simulink model "Tesis_Rectificador_Controlador_Observador_04"  (R2012b)
settings: Solver=ode1  StartTime=0.0  StopTime=1.0  FixedStep=1e-5/6  RelTol=1e-3
libraries: simulink x1
settings Model: Creator=Ramm  LastModifiedBy=Ramm

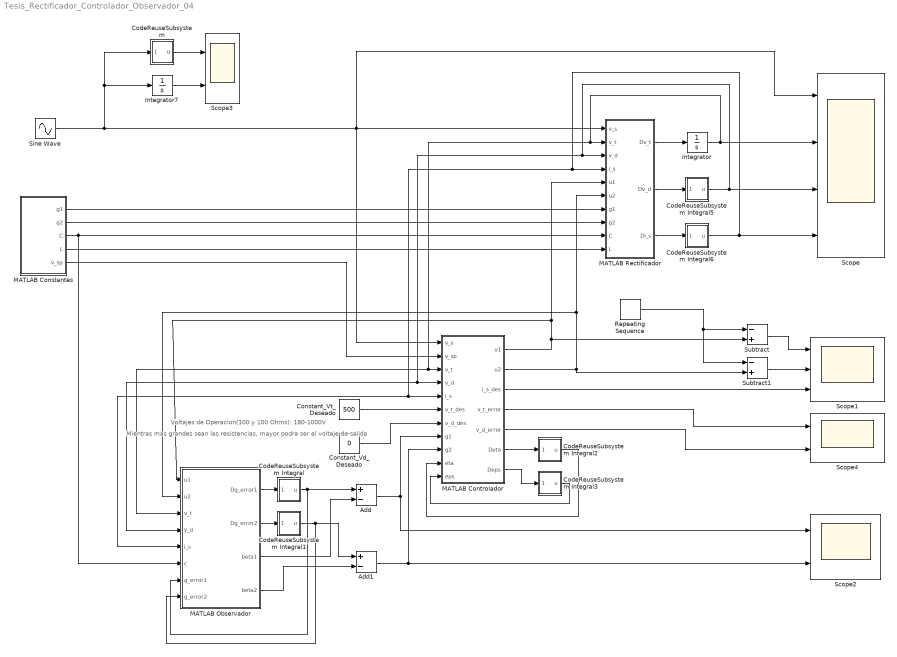
== system Tesis_Rectificador_Controlador_Observador_04 ==
  note: Mientras mas grandes sean las resistencias,
      | mayor podra ser el voltaje de salida
  note: Voltajes de Operacion(100 y 100 Ohms): 180-1000V
  Add : Sum  Inputs=+-
  Add1 : Sum  Inputs=+-
  CodeReuseSubsystem : Subsystem  TreatAsAtomicUnit=on
      settings: RTWFcnNameOpts=Use subsystem name  RTWFileNameOpts=Use function name
  CodeReuseSubsystem Integral : Subsystem  TreatAsAtomicUnit=on
      settings: RTWFcnNameOpts=Use subsystem name  RTWFileNameOpts=Use function name
  CodeReuseSubsystem Integral1 : Subsystem  TreatAsAtomicUnit=on
      settings: RTWFcnNameOpts=Use subsystem name  RTWFileNameOpts=Use function name
  CodeReuseSubsystem Integral2 : Subsystem  TreatAsAtomicUnit=on
      settings: RTWFcnNameOpts=Use subsystem name  RTWFileNameOpts=Use function name
  CodeReuseSubsystem Integral3 : Subsystem  TreatAsAtomicUnit=on
      settings: RTWFcnNameOpts=Use subsystem name  RTWFileNameOpts=Use function name
  CodeReuseSubsystem Integral5 : Subsystem  TreatAsAtomicUnit=on
      settings: RTWFcnNameOpts=Use subsystem name  RTWFileNameOpts=Use function name
  CodeReuseSubsystem Integral6 : Subsystem  TreatAsAtomicUnit=on
      settings: RTWFcnNameOpts=Use subsystem name  RTWFileNameOpts=Use function name
  Constant_Vd_Deseado : Constant  Value=0
  Constant_Vt_Deseado : Constant  Value=500
  Integrator : Integrator
  Integrator7 : Integrator  InitialCondition=0.02
  "MATLAB Constantes " : MATLAB Function  TreatAsAtomicUnit=on
  MATLAB Controlador : MATLAB Function  TreatAsAtomicUnit=on
  "MATLAB Observador " : MATLAB Function  TreatAsAtomicUnit=on
  "MATLAB Rectificador " : MATLAB Function  TreatAsAtomicUnit=on
  Repeating Sequence : simulink/Sources/Repeating Sequence  rep_seq_t=[0 1.655e-5]  rep_seq_y=[0 1]
  Scope : Scope  NumInputPorts=4
      settings: TimeRange=0.5  YMin=-200~425~-1.525~-30  YMax=200~600~-1.325~25
  Scope1 : Scope  NumInputPorts=3
      settings: TimeRange=1  YMin=-350~-350~-1.5  YMax=350~350~1.5
  Scope2 : Scope  NumInputPorts=2
      settings: TimeRange=0.7000000000000001  YMin=-0.002~-0.005  YMax=0.012~0.02  SaveName=ScopeData3
  Scope3 : Scope  NumInputPorts=2
      settings: YMin=-5~-5  YMax=5~5  SaveName=ScopeData4
  Scope4 : Scope  NumInputPorts=2
      settings: YMin=-129~-1.035  YMax=-118~-0.945  SaveName=ScopeData2
  Sine Wave : Sin  Amplitude=180  Frequency=120*pi  SampleTime=0
  Subtract : Sum  Inputs=-+
  Subtract1 : Sum  Inputs=-+
  wires:
  Constant_Vt_Deseado/1 -> MATLAB Controlador/6(v_t_des)
  Constant_Vd_Deseado/1 -> MATLAB Controlador/7(v_d_des)
  "MATLAB Observador "/1(Dg_error1) -> CodeReuseSubsystem Integral/1(Du)
  CodeReuseSubsystem Integral/1(u) -> "MATLAB Observador "/7(g_error1), Add/1
  Add/1 -> Scope2/1, MATLAB Controlador/8(g1)
  Add1/1 -> MATLAB Controlador/9(g2), Scope2/2
  MATLAB Controlador/6(Deta) -> CodeReuseSubsystem Integral2/1(Du)
  MATLAB Controlador/7(Deps) -> CodeReuseSubsystem Integral3/1(Du)
  CodeReuseSubsystem Integral2/1(u) -> MATLAB Controlador/10(eta)
  CodeReuseSubsystem Integral3/1(u) -> MATLAB Controlador/11(eps)
  "MATLAB Constantes "/1(g1) -> "MATLAB Rectificador "/7(g1)
  "MATLAB Constantes "/2(g2) -> "MATLAB Rectificador "/8(g2)
  "MATLAB Constantes "/3(C) -> "MATLAB Observador "/6(c), "MATLAB Rectificador "/9(C)
  "MATLAB Constantes "/4(L) -> "MATLAB Rectificador "/10(L)
  "MATLAB Constantes "/5(v_sp) -> MATLAB Controlador/2(v_sp)
  Sine Wave/1 -> CodeReuseSubsystem/1(Du), Integrator7/1, Scope/1, MATLAB Controlador/1(v_s), "MATLAB Rectificador "/1(v_s)
  "MATLAB Rectificador "/1(Dv_t) -> Integrator/1
  "MATLAB Rectificador "/2(Dv_d) -> CodeReuseSubsystem Integral5/1(Du)
  "MATLAB Rectificador "/3(Di_s) -> CodeReuseSubsystem Integral6/1(Du)
  MATLAB Controlador/1(u1) -> Subtract/2, "MATLAB Observador "/1(u1), "MATLAB Rectificador "/5(u1)
  Integrator/1 -> Scope/2, "MATLAB Observador "/3(v_t), MATLAB Controlador/3(v_t), "MATLAB Rectificador "/2(v_t)
  CodeReuseSubsystem Integral5/1(u) -> Scope/3, MATLAB Controlador/4(v_d), "MATLAB Observador "/4(v_d), "MATLAB Rectificador "/3(v_d)
  CodeReuseSubsystem Integral6/1(u) -> Scope/4, "MATLAB Observador "/5(i_s), MATLAB Controlador/5(i_s), "MATLAB Rectificador "/4(i_s)
  MATLAB Controlador/4(v_t_error) -> Scope4/1
  MATLAB Controlador/5(v_d_error) -> Scope4/2
  MATLAB Controlador/3(i_s_des) -> Scope1/3
  "MATLAB Observador "/3(beta1) -> Add/2
  "MATLAB Observador "/2(Dg_error2) -> CodeReuseSubsystem Integral1/1(Du)
  CodeReuseSubsystem Integral1/1(u) -> "MATLAB Observador "/8(g_error2), Add1/1
  "MATLAB Observador "/4(beta2) -> Add1/2
  MATLAB Controlador/2(u2) -> "MATLAB Rectificador "/6(u2), "MATLAB Observador "/2(u2), Subtract1/2
  Subtract1/1 -> Scope1/2
  Subtract/1 -> Scope1/1
  Repeating Sequence/1 -> Subtract/1, Subtract1/1
  CodeReuseSubsystem/1(u) -> Scope3/1
  Integrator7/1 -> Scope3/2

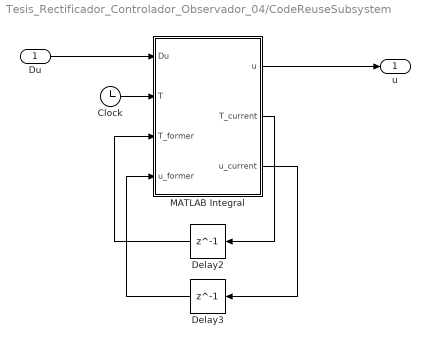
== system Tesis_Rectificador_Controlador_Observador_04/CodeReuseSubsystem ==
  Du : Inport
  Clock : Clock
  Delay2 : Delay  DelayLength=1  InitialCondition=0
  Delay3 : Delay  DelayLength=1  InitialCondition=0
  MATLAB Integral : MATLAB Function  TreatAsAtomicUnit=on
  u : Outport
  wires:
  Clock/1 -> MATLAB Integral/2(T)
  Du/1 -> MATLAB Integral/1(Du)
  MATLAB Integral/1(u) -> u/1
  Delay3/1 -> MATLAB Integral/4(u_former)
  MATLAB Integral/3(u_current) -> Delay3/1
  Delay2/1 -> MATLAB Integral/3(T_former)
  MATLAB Integral/2(T_current) -> Delay2/1

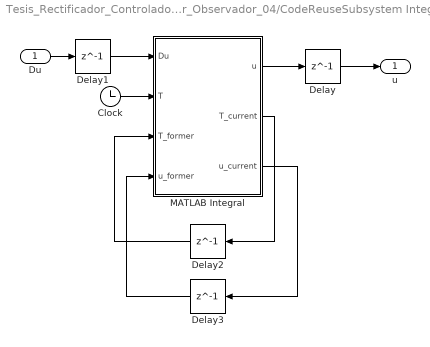
== system Tesis_Rectificador_Controlador_Observador_04/CodeReuseSubsystem Integral ==
  Du : Inport
  Clock : Clock
  Delay{,1..3} (4 alike) : Delay  DelayLength=1  InitialCondition=0
  MATLAB Integral : MATLAB Function  TreatAsAtomicUnit=on
  u : Outport
  wires:
  MATLAB Integral/2(T_current) -> Delay2/1
  Delay2/1 -> MATLAB Integral/3(T_former)
  MATLAB Integral/3(u_current) -> Delay3/1
  Delay3/1 -> MATLAB Integral/4(u_former)
  Clock/1 -> MATLAB Integral/2(T)
  MATLAB Integral/1(u) -> Delay/1
  Delay/1 -> u/1
  Du/1 -> Delay1/1
  Delay1/1 -> MATLAB Integral/1(Du)

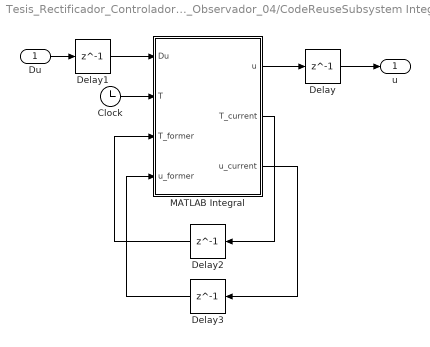
== system Tesis_Rectificador_Controlador_Observador_04/CodeReuseSubsystem Integral1 ==
  Du : Inport
  Clock : Clock
  Delay{,1..3} (4 alike) : Delay  DelayLength=1  InitialCondition=0
  MATLAB Integral : MATLAB Function  TreatAsAtomicUnit=on
  u : Outport
  wires:
  Delay1/1 -> MATLAB Integral/1(Du)
  Du/1 -> Delay1/1
  Delay/1 -> u/1
  MATLAB Integral/1(u) -> Delay/1
  Clock/1 -> MATLAB Integral/2(T)
  Delay3/1 -> MATLAB Integral/4(u_former)
  MATLAB Integral/3(u_current) -> Delay3/1
  Delay2/1 -> MATLAB Integral/3(T_former)
  MATLAB Integral/2(T_current) -> Delay2/1

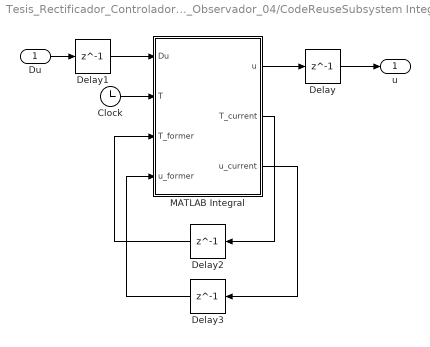
== system Tesis_Rectificador_Controlador_Observador_04/CodeReuseSubsystem Integral2 ==
  Du : Inport
  Clock : Clock
  Delay{,1..3} (4 alike) : Delay  DelayLength=1  InitialCondition=0
  MATLAB Integral : MATLAB Function  TreatAsAtomicUnit=on
  u : Outport
  wires:
  MATLAB Integral/2(T_current) -> Delay2/1
  Delay2/1 -> MATLAB Integral/3(T_former)
  MATLAB Integral/3(u_current) -> Delay3/1
  Delay3/1 -> MATLAB Integral/4(u_former)
  Clock/1 -> MATLAB Integral/2(T)
  MATLAB Integral/1(u) -> Delay/1
  Delay/1 -> u/1
  Du/1 -> Delay1/1
  Delay1/1 -> MATLAB Integral/1(Du)

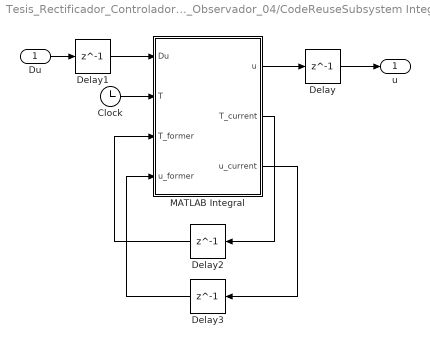
== system Tesis_Rectificador_Controlador_Observador_04/CodeReuseSubsystem Integral3 ==
  Du : Inport
  Clock : Clock
  Delay{,1..3} (4 alike) : Delay  DelayLength=1  InitialCondition=0
  MATLAB Integral : MATLAB Function  TreatAsAtomicUnit=on
  u : Outport
  wires:
  Delay1/1 -> MATLAB Integral/1(Du)
  Du/1 -> Delay1/1
  Delay/1 -> u/1
  MATLAB Integral/1(u) -> Delay/1
  Clock/1 -> MATLAB Integral/2(T)
  Delay3/1 -> MATLAB Integral/4(u_former)
  MATLAB Integral/3(u_current) -> Delay3/1
  Delay2/1 -> MATLAB Integral/3(T_former)
  MATLAB Integral/2(T_current) -> Delay2/1

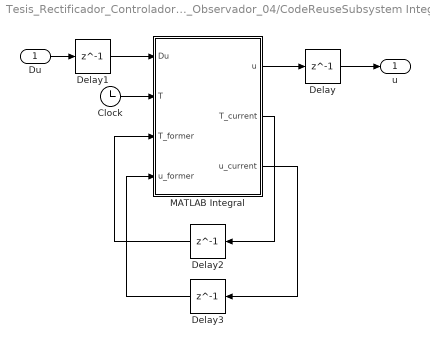
== system Tesis_Rectificador_Controlador_Observador_04/CodeReuseSubsystem Integral5 ==
  Du : Inport
  Clock : Clock
  Delay : Delay  DelayLength=1  InitialCondition=1
  Delay1 : Delay  DelayLength=1  InitialCondition=0
  Delay2 : Delay  DelayLength=1  InitialCondition=0
  Delay3 : Delay  DelayLength=1  InitialCondition=0
  MATLAB Integral : MATLAB Function  TreatAsAtomicUnit=on
  u : Outport
  wires:
  Delay1/1 -> MATLAB Integral/1(Du)
  Du/1 -> Delay1/1
  Delay/1 -> u/1
  MATLAB Integral/1(u) -> Delay/1
  Clock/1 -> MATLAB Integral/2(T)
  Delay3/1 -> MATLAB Integral/4(u_former)
  MATLAB Integral/3(u_current) -> Delay3/1
  Delay2/1 -> MATLAB Integral/3(T_former)
  MATLAB Integral/2(T_current) -> Delay2/1

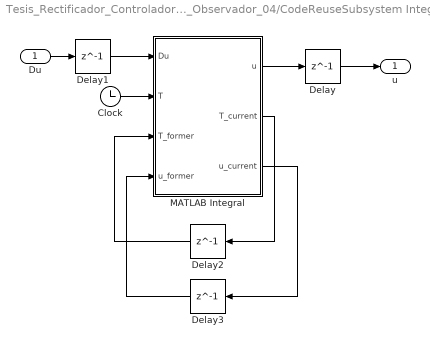
== system Tesis_Rectificador_Controlador_Observador_04/CodeReuseSubsystem Integral6 ==
  Du : Inport
  Clock : Clock
  Delay : Delay  DelayLength=1  InitialCondition=1
  Delay1 : Delay  DelayLength=1  InitialCondition=0
  Delay2 : Delay  DelayLength=1  InitialCondition=0
  Delay3 : Delay  DelayLength=1  InitialCondition=0
  MATLAB Integral : MATLAB Function  TreatAsAtomicUnit=on
  u : Outport
  wires:
  MATLAB Integral/2(T_current) -> Delay2/1
  Delay2/1 -> MATLAB Integral/3(T_former)
  MATLAB Integral/3(u_current) -> Delay3/1
  Delay3/1 -> MATLAB Integral/4(u_former)
  Clock/1 -> MATLAB Integral/2(T)
  MATLAB Integral/1(u) -> Delay/1
  Delay/1 -> u/1
  Du/1 -> Delay1/1
  Delay1/1 -> MATLAB Integral/1(Du)

== matlab function Tesis_Rectificador_Controlador_Observador_04/MATLAB Controlador ==
  data: v_s input; v_sp input; u1 output; v_t input; v_d input; i_s input; v_t_des input; v_d_des input; g1 input; g2 input; u2 output; i_s_des output; v_t_error output; v_d_error output; Deta output; Deps output; eta input; eps input
function [u1, u2, i_s_des, v_t_error, v_d_error, Deta, Deps] = fcn(v_s, v_sp, v_t, v_d, i_s, v_t_des, v_d_des, g1, g2, eta, eps)
%#codegen
%Constantes de proporcionalidad -----------------------------------
k = 10000;%Se encarga de disminuir el error de la corriente, mientras mas grande sea mas rapido decaera el error, pero puede volverse inestable

%Para la corriente deseada
kp1 = 1e-2;%1e-2;%Debe ser muy chico para ver el observador pero deja de controlar(Oscilatorio (v_t))
ki1 = 10;%1e-2;%Debe ser muy chico para ver el observador pero deja de controlar(Compensacion de estado estable(v_t))

%Señales de control
kp2 = 250;%250;
ki2 = 500;%500;

%*****************************************************************************************************************************
%Calculos previos-------------------------------------------------
v_t_error = v_t - v_t_des;
i_s_des = -((v_s*v_t)/(2*v_sp*v_sp))*(-g1*v_t -g2*v_d + kp1*v_t_error +ki1*eta);
i_s_error = i_s - i_s_des;
v_d_error = v_d - v_d_des;

%Salidas-------------------------------------------------

%Con los despejes hechos previamente a mano
u1_v = -(1/v_t)*sign(i_s)*(v_s + k*i_s_error) + (i_s_des/(2+2*i_s_des*i_s_des))*(-g2*v_t -g1*v_d +kp2*v_d_error + ki2*eps) + 1;
if(u1_v > 1)%Solo evita que se pase de 1 y 0, pero los valores intermedios permanecen
    u1 = 1;
elseif(u1_v <0)
    u1 = 0;
else
    u1 = u1_v;
end

u2_v= -(1/v_t)*sign(i_s)*(v_s + k*i_s_error) - (i_s_des/(2+2*i_s_des*i_s_des))*(-g2*v_t -g1*v_d +kp2*v_d_error + ki2*eps) + 1;
if(u2_v > 1)
    u2 = 1;
elseif(u2_v <0)
    u2 = 0;
else
    u2 = u2_v;
end

Deta = v_t_error;
Deps = v_d_error;

== matlab function Tesis_Rectificador_Controlador_Observador_04/MATLAB Rectificador  ==
  data: v_s input; v_t input; v_d input; i_s input; Dv_t output; u1 input; u2 input; Dv_d output; Di_s output; g1 input; g2 input; C input; L input
function [Dv_t, Dv_d, Di_s] = fcn(v_s, v_t, v_d, i_s, u1, u2, g1, g2, C, L)
%#codegen

%Salidas del circuito Rectificador
Dv_t = (-v_t*g1 -v_d*g2 +i_s*sign(i_s)*(2-u1-u2))/C;
Dv_d = (-v_t*g2 -v_d*g1 + i_s*(u2-u1))/C;
Di_s = (-0.5*sign(i_s)*v_t*(2 -u1 -u2) -0.5*v_d*(u2-u1) + v_s)/L;

== matlab function Tesis_Rectificador_Controlador_Observador_04/CodeReuseSubsystem/MATLAB Integral ==
  data: u output; T_current output; u_current output; Du input; T input; T_former input; u_former input
function [u, T_current, u_current] = fcn(Du, T, T_former, u_former)
%#codegen
T_current = T;
u = Du*(T_current - T_former) + u_former;
u_current = u;

== matlab function Tesis_Rectificador_Controlador_Observador_04/MATLAB Constantes  ==
  data: g1 output; g2 output; C output; L output; v_sp output
function [g1, g2, C, L, v_sp] = fcn()
%#codegen
r1 = 100;%100
r2 = 100;%100

v_sp = 180;
C = 470e-6;
L = 10e-3;
g1=(1/(2*r1))+(1/(2*r2));
g2=(1/(2*r1))-(1/(2*r2));

== matlab function Tesis_Rectificador_Controlador_Observador_04/MATLAB Observador  ==
  data: u1 input; Dg_error1 output; u2 input; v_t input; v_d input; i_s input; c input; g_error1 input; Dg_error2 output; beta1 output; beta2 output; g_error2 input
function [Dg_error1, Dg_error2, beta1, beta2] = fcn(u1, u2, v_t, v_d, i_s,  c, g_error1, g_error2)
%#codegen

%Constantes------------------------------------------
gamma1 = 100e-5;
gamma2 = 100e-5;

%Matrices necesarias---------------------------------
gamma = [gamma1, 0; 0, gamma2];
Gv = [v_t, v_d; v_d, v_t];
F_is = [i_s*sign(i_s)*(2 -u1 -u2); i_s*(u2 -u1)];
g_error = [g_error1; g_error2];

%%Calculos intermedios-------------------------------
Dbeta = c*gamma*Gv;
beta = c*gamma*[(v_t*v_t + v_d*v_d)/2; v_t*v_d];

%Ecuacion matricial governante-----------------------
Dg_error = Dbeta*(1/c)*(F_is - Gv*(g_error - beta));

%Salidas---------------------------------------------
Dg_error1 = Dg_error(1);
Dg_error2 = Dg_error(2);
beta1 = beta(1);
beta2 = beta(2);

== matlab function Tesis_Rectificador_Controlador_Observador_04/CodeReuseSubsystem Integral/MATLAB Integral ==
  data: u output; T_current output; u_current output; Du input; T input; T_former input; u_former input
function [u, T_current, u_current] = fcn(Du, T, T_former, u_former)
%#codegen
T_current = T;
u = Du*(T_current - T_former) + u_former;
u_current = u;

== matlab function Tesis_Rectificador_Controlador_Observador_04/CodeReuseSubsystem Integral1/MATLAB Integral ==
  data: u output; T_current output; u_current output; Du input; T input; T_former input; u_former input
function [u, T_current, u_current] = fcn(Du, T, T_former, u_former)
%#codegen
T_current = T;
u = Du*(T_current - T_former) + u_former;
u_current = u;

== matlab function Tesis_Rectificador_Controlador_Observador_04/CodeReuseSubsystem Integral2/MATLAB Integral ==
  data: u output; T_current output; u_current output; Du input; T input; T_former input; u_former input
function [u, T_current, u_current] = fcn(Du, T, T_former, u_former)
%#codegen
T_current = T;
u = Du*(T_current - T_former) + u_former;
u_current = u;

== matlab function Tesis_Rectificador_Controlador_Observador_04/CodeReuseSubsystem Integral3/MATLAB Integral ==
  data: u output; T_current output; u_current output; Du input; T input; T_former input; u_former input
function [u, T_current, u_current] = fcn(Du, T, T_former, u_former)
%#codegen
T_current = T;
u = Du*(T_current - T_former) + u_former;
u_current = u;

== matlab function Tesis_Rectificador_Controlador_Observador_04/CodeReuseSubsystem Integral5/MATLAB Integral ==
  data: u output; T_current output; u_current output; Du input; T input; T_former input; u_former input
function [u, T_current, u_current] = fcn(Du, T, T_former, u_former)
%#codegen
T_current = T;
u = Du*(T_current - T_former) + u_former;
u_current = u;

== matlab function Tesis_Rectificador_Controlador_Observador_04/CodeReuseSubsystem Integral6/MATLAB Integral ==
  data: u output; T_current output; u_current output; Du input; T input; T_former input; u_former input
function [u, T_current, u_current] = fcn(Du, T, T_former, u_former)
%#codegen
T_current = T;
u = Du*(T_current - T_former) + u_former;
u_current = u;
